simulink model "SUPERVISOR_SEGURIDAD"  (R2024b)
settings: Solver=VariableStepAuto  StartTime=0.0  StopTime=10.0  RelTol=1e-3
settings Model: Creator=ribei  LastModifiedBy=ribei

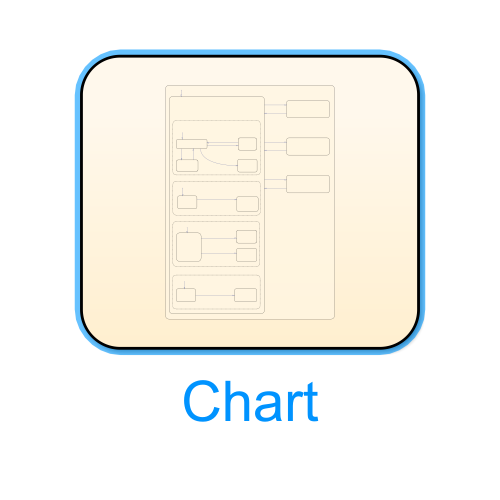
[thumbnail: Simulink's stored preview of the top-level diagram]
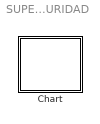
== system SUPERVISOR_SEGURIDAD ==
  Chart : Stateflow chart  TreatAsAtomicUnit=on

== stateflow chart SUPERVISOR_SEGURIDAD/Chart ==
  state NIVEL_0
    state VERIFY
      entry:
      emergency=0;
      BRK_t=1;
      BRK_h=1;
      BRK_hE=1;
      n=0;
      state Watchdog [parallel]
        entry:
        n=0;
        settings: executionOrder=1
        state Alive
          entry:
          n=0;
        state StandBy
        state Reset
          entry:
          emergency=1;
          type=0;
        state Sum
          entry:
          n=n+1
        (default) -> NIVEL_0.VERIFY.Watchdog.StandBy
        Alive -> NIVEL_0.VERIFY.Watchdog.StandBy : [Alive==1]
        NIVEL_0.VERIFY.Watchdog.StandBy -> Alive [order 1] : [true]
        NIVEL_0.VERIFY.Watchdog.StandBy -> Sum [order 2] : after(1,sec)
        Sum -> NIVEL_0.VERIFY.Watchdog.StandBy : [true]
        NIVEL_0.VERIFY.Watchdog.StandBy -> Reset [order 3] : [n>=5]
      state HSE [parallel]
        settings: executionOrder=2
        state StandBy
        state HS
          entry:
          emergency=1;
          type=0;
        (default) -> NIVEL_0.VERIFY.HSE.StandBy
        NIVEL_0.VERIFY.HSE.StandBy -> HS : [HSE==0]
      state FCE [parallel]
        settings: executionOrder=3
        state Carro
          entry:
          emergency=1;
          type=1;
        state StandBy
        state Izaje
          entry:
          emergency=1;
          type=2;
        (default) -> NIVEL_0.VERIFY.FCE.StandBy
        NIVEL_0.VERIFY.FCE.StandBy -> Carro [order 2] : [FCE_IZQ||FCE_DER]
        NIVEL_0.VERIFY.FCE.StandBy -> Izaje [order 1] : [FCE_SUP||FCE_INF]
      state SOBREVELOCIDAD [parallel]
        settings: executionOrder=4
        state SobreVel
          entry:
          emergency=1;
          type=2;
        state StandBy
        (default) -> NIVEL_0.VERIFY.SOBREVELOCIDAD.StandBy
        NIVEL_0.VERIFY.SOBREVELOCIDAD.StandBy -> SobreVel : [dl_hm>=1.2*dl_hm_max]
    state Type0
      entry:
      BRK_t=0;
      BRK_h=0;
      BRK_hE=0;
    state Type1
      entry:
      BRK_t=0;
    state Type2
      entry:
      BRK_h=0;
      BRK_hE=0;
    (default) -> VERIFY
    VERIFY -> Type0 [order 1] : [type==0]
    Type0 -> VERIFY : [norm]
    VERIFY -> Type1 [order 2] : [type==1]
    Type1 -> VERIFY : [norm]
    VERIFY -> Type2 [order 3] : [type==2]
    Type2 -> VERIFY : [norm]
